simulink model "Modified_CR"  (R2014b)
settings: Solver=ode45  StartTime=0.0  StopTime=10  RelTol=1e-3
undefined symbols (not defined in the file or in its folder): A, B, C, D
settings Model: Creator=uidd7441  LastModifiedBy=uidd7441

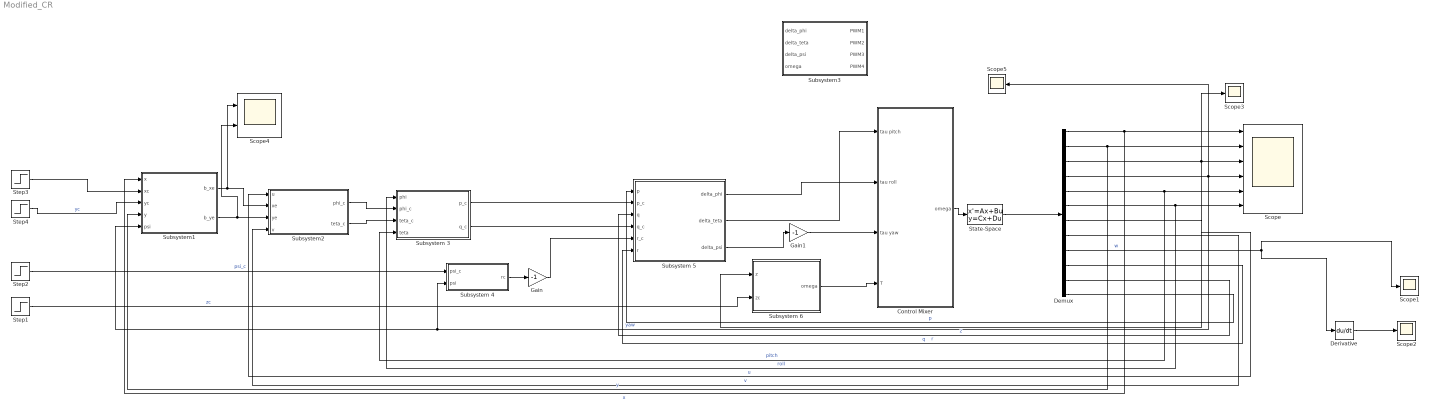
== system Modified_CR ==
  Control Mixer : Subsystem  AncestorBlock=roblocks/Dynamics/Control Mixer 4
      mask help: Quadrotor control mixer
      mask Help:
      | Determine rotor speeds based on desired torques and thrust.
      | 
      | <b>Inputs::</b>
      | 
      | tau pitch (1x1)  desired pitching torque [Nm]
      | tau roll (1x1)   desired rolling torque [Nm]
      | tau yaw (1x1)    desired yawing torque [Nm]
      | T (1x1)          desired thrust [N]
      | 
      | <b>Outputs::</b>
      | 
      | w1 (1x1) angular velocity of rotor 1 [rad]
      | w2 (1x1) angular velocity of rotor 2 [rad]
      | w3 (1x1) angular velocity of rotor 3 [rad]
      | w4 (1x1) angular velocity of rotor 4 [rad]
      | 
      | <b>Notes::</b>
      | 
      | - Assumes the rotor labelling convention of RVC Fig 4.16.
      | - The quadrotor is underactuated and has only 4 inputs.
  Demux : Demux  Outputs=12
  Derivative : Derivative
  Gain : Gain  Gain=-1
  Gain1 : Gain  Gain=-1
  Scope : Scope  NumInputPorts=6
      settings: YMin=0~0~0~0~0~-4e+06  YMax=2e+08~2e+08~1000~400000~4e+06~0
  Scope{1..3,5} (4 alike) : Scope
      Scope2 settings: SaveName=ScopeData2
      Scope3 settings: SaveName=ScopeData3
      Scope5 settings: TimeRange=2.494596015329648  YMin=250000  YMax=450000  SaveName=ScopeData5  MaxDataPoints=5000000
  Scope4 : Scope  NumInputPorts=2
      settings: YMin=-5~-5  YMax=5~5  SaveName=ScopeData10
  State-Space : StateSpace  A=A  B=B  C=C  D=D  X0=[0 0 0 0 0 0 0 0 0 0 0 0]'
  Step1 : Step  Time=0  SampleTime=0
  Step2 : Step  Time=0  After=60  SampleTime=0
  Step3 : Step  Time=0  SampleTime=0
  Step4 : Step  Time=0  SampleTime=0
  Subsystem 3 : Subsystem
  Subsystem 4 : Subsystem
  Subsystem 5 : Subsystem
  Subsystem 6 : Subsystem
  Subsystem1 : Subsystem
  Subsystem2 : Subsystem
  Subsystem3 : Subsystem
  wires:
  Step1/1 -> Subsystem 6/2(zc)  "zc"
  Step4/1 -> Subsystem1/3(yc)  "yc"
  Step2/1 -> Subsystem 4/1(psi_c)  "psi_c"
  Subsystem1/2(b_ye) -> Scope4/2, Subsystem2/3(ye)
  Subsystem 4/1(rc) -> Gain/1
  Subsystem 6/1(omega) -> Control Mixer/4(T)
  State-Space/1 -> Demux/1
  Subsystem1/1(b_xe) -> Scope4/1, Subsystem2/2(xe)
  Step3/1 -> Subsystem1/2(xc)
  Demux/3 -> Subsystem 6/1(z), Scope3/1, Scope/3  "z"
  Demux/1 -> Subsystem1/1(x), Scope/1  "x"
  Demux/2 -> Subsystem1/4(y), Scope/2  "y"
  Demux/4 -> Subsystem1/5(psi), Subsystem 4/2(psi), Scope5/1, Scope/4  "yaw"
  Demux/5 -> Subsystem 3/4(teta), Scope/5  "pitch"
  Demux/6 -> Subsystem 3/1("phi "), Scope/6  "roll"
  Demux/7 -> Subsystem2/1(u)  "u"
  Demux/8 -> Subsystem2/4(v)  "v"
  Demux/9 -> Scope1/1, Derivative/1  "w"
  Demux/11 -> Subsystem 5/3(q)  "q"
  Demux/12 -> Subsystem 5/1(p)  "p"
  Demux/10 -> Subsystem 5/6(r)  "r"
  Derivative/1 -> Scope2/1
  Subsystem 5/3(delta_psi) -> Gain1/1
  Subsystem 3/1(p_c) -> Subsystem 5/2(p_c)
  Subsystem 3/2(q_c) -> Subsystem 5/4(q_c)
  Gain/1 -> Subsystem 5/5(r_c)
  Gain1/1 -> Control Mixer/3(tau yaw)
  Control Mixer/1(omega) -> State-Space/1
  Subsystem2/1(phi_c) -> Subsystem 3/2(phi_c)
  Subsystem2/2(teta_c) -> Subsystem 3/3(teta_c)
  Subsystem 5/1(delta_phi) -> Control Mixer/2(tau roll)
  Subsystem 5/2(delta_teta) -> Control Mixer/1(tau pitch)

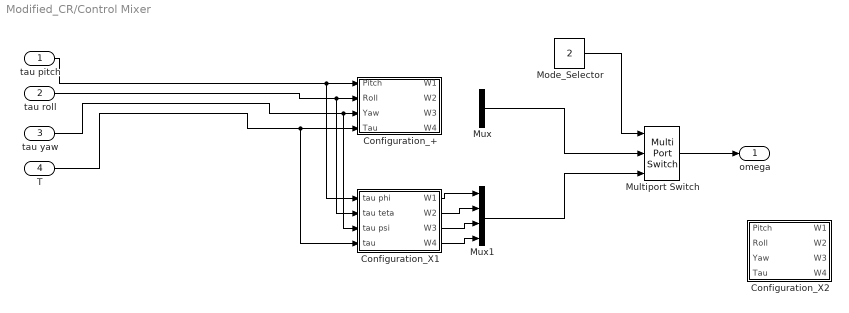
== system Modified_CR/Control Mixer ==
  tau pitch : Inport
  tau roll : Inport  Port=2
  tau yaw : Inport  Port=3
  T : Inport  Port=4
  Configuration_+ : Subsystem
  Configuration_X1 : Subsystem
  Configuration_X2 : Subsystem
  Mode_Selector : Constant  Value=2
  Multiport Switch : MultiPortSwitch  Inputs=2
  Mux : Mux
  Mux1 : Mux
  omega : Outport
  wires:
  Mux/1 -> Multiport Switch/2
  Multiport Switch/1 -> omega/1
  Mode_Selector/1 -> Multiport Switch/1
  T/1 -> Configuration_X1/4(tau), Configuration_+/4(Tau)
  tau yaw/1 -> Configuration_X1/3(tau psi), Configuration_+/3(Yaw)
  tau roll/1 -> Configuration_X1/2(tau teta), Configuration_+/2(Roll)
  tau pitch/1 -> Configuration_X1/1(tau phi), Configuration_+/1(Pitch)
  Mux1/1 -> Multiport Switch/3
  Configuration_X1/4(W4) -> Mux1/4
  Configuration_X1/3(W3) -> Mux1/3
  Configuration_X1/2(W2) -> Mux1/2
  Configuration_X1/1(W1) -> Mux1/1

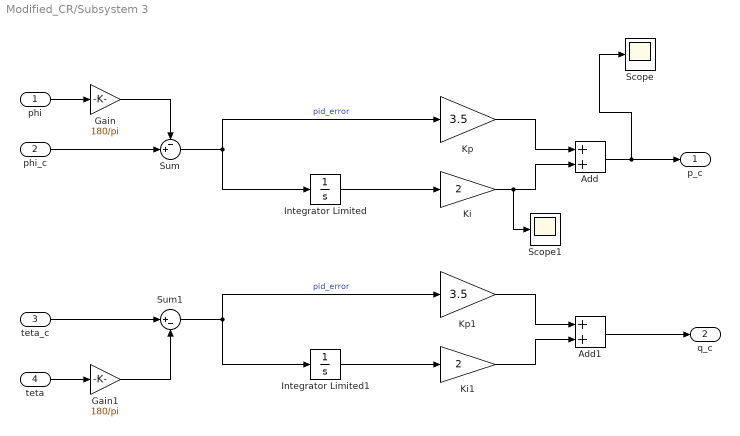
== system Modified_CR/Subsystem 3 ==
  "phi " : Inport
  phi_c : Inport  Port=2
  teta_c : Inport  Port=3
  teta : Inport  Port=4
  Add : Sum
  Add1 : Sum
  Gain : Gain  Gain=180/pi
  Gain1 : Gain  Gain=180/pi
  Integrator Limited : Integrator  LimitOutput=on  UpperSaturationLimit=20  LowerSaturationLimit=-20
  Integrator Limited1 : Integrator  LimitOutput=on  UpperSaturationLimit=20  LowerSaturationLimit=-20
  Ki : Gain  Gain=2  OutMin=[-200]  OutMax=[200]
  Ki1 : Gain  Gain=2  OutMin=[-200]  OutMax=[200]
  Kp : Gain  Gain=3.5  OutMin=[-200]  OutMax=[200]
  Kp1 : Gain  Gain=3.5  OutMin=[-200]  OutMax=[200]
  Scope : Scope
      settings: SaveName=ScopeData7
  Scope1 : Scope
      settings: SaveName=ScopeData8
  Sum : Sum  Inputs=-+|
  Sum1 : Sum  Inputs=|+-
  p_c : Outport
  q_c : Outport  Port=2
  wires:
  "phi "/1 -> Gain/1
  phi_c/1 -> Sum/2
  teta_c/1 -> Sum1/1
  teta/1 -> Gain1/1
  Add/1 -> Scope/1, p_c/1
  Add1/1 -> q_c/1
  Sum/1 -> Integrator Limited/1, Kp/1  "pid_error"
  Integrator Limited/1 -> Ki/1
  Kp/1 -> Add/1
  Sum1/1 -> Integrator Limited1/1, Kp1/1  "pid_error"
  Integrator Limited1/1 -> Ki1/1
  Kp1/1 -> Add1/1
  Ki1/1 -> Add1/2
  Gain/1 -> Sum/1
  Gain1/1 -> Sum1/2
  Ki/1 -> Scope1/1, Add/2

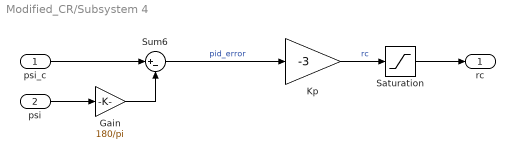
== system Modified_CR/Subsystem 4 ==
  psi_c : Inport
  psi : Inport  Port=2
  Gain : Gain  Gain=180/pi
  Kp : Gain  Gain=-3  OutMin=[-200]  OutMax=[200]
  Saturation : Saturate  UpperLimit=200  LowerLimit=-200
  Sum6 : Sum  Inputs=|+-
  rc : Outport
  wires:
  Kp/1 -> Saturation/1  "rc"
  psi_c/1 -> Sum6/1
  psi/1 -> Gain/1
  Sum6/1 -> Kp/1  "pid_error"
  Saturation/1 -> rc/1
  Gain/1 -> Sum6/2

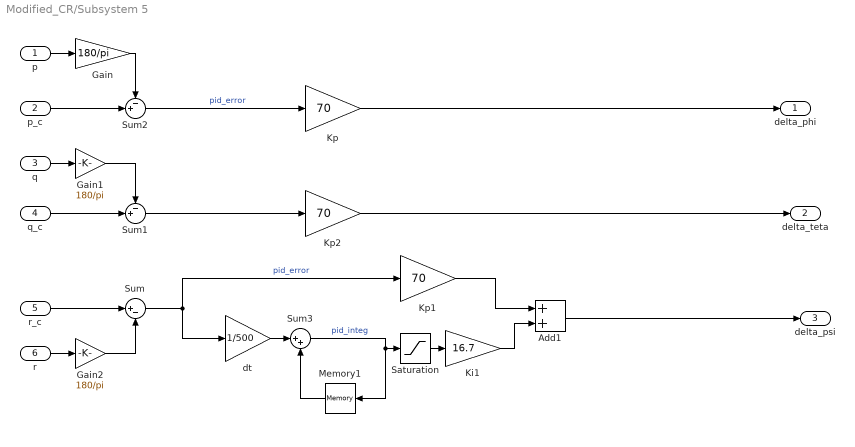
== system Modified_CR/Subsystem 5 ==
  p : Inport
  p_c : Inport  Port=2
  q : Inport  Port=3
  q_c : Inport  Port=4
  r_c : Inport  Port=5
  r : Inport  Port=6
  Add1 : Sum
  Gain : Gain  Gain=180/pi
  Gain1 : Gain  Gain=180/pi
  Gain2 : Gain  Gain=180/pi
  Ki1 : Gain  Gain=16.7  OutMin=[-200]  OutMax=[200]
  Kp : Gain  Gain=70  OutMin=[-200]  OutMax=[200]
  Kp1 : Gain  Gain=70  OutMin=[-200]  OutMax=[200]
  Kp2 : Gain  Gain=70  OutMin=[-200]  OutMax=[200]
  Memory1 : Memory
  Saturation : Saturate  UpperLimit=166.7  LowerLimit=-166.7
  Sum : Sum  Inputs=|+-
  Sum1 : Sum  Inputs=-+|
  Sum2 : Sum  Inputs=-+|
  Sum3 : Sum  Inputs=|++
  dt : Gain  Gain=1/500  OutMin=[-200]  OutMax=[200]
  delta_phi : Outport
  delta_teta : Outport  Port=2
  delta_psi : Outport  Port=3
  wires:
  q/1 -> Gain1/1
  q_c/1 -> Sum1/2
  p_c/1 -> Sum2/2
  p/1 -> Gain/1
  r_c/1 -> Sum/1
  r/1 -> Gain2/1
  Sum1/1 -> Kp2/1
  Kp/1 -> delta_phi/1
  Kp2/1 -> delta_teta/1
  Add1/1 -> delta_psi/1
  Sum2/1 -> Kp/1  "pid_error"
  Kp1/1 -> Add1/1
  Ki1/1 -> Add1/2
  dt/1 -> Sum3/1
  Sum/1 -> Kp1/1, dt/1  "pid_error"
  Sum3/1 -> Saturation/1, Memory1/1  "pid_integ"
  Memory1/1 -> Sum3/2
  Saturation/1 -> Ki1/1
  Gain/1 -> Sum2/1
  Gain1/1 -> Sum1/1
  Gain2/1 -> Sum/2

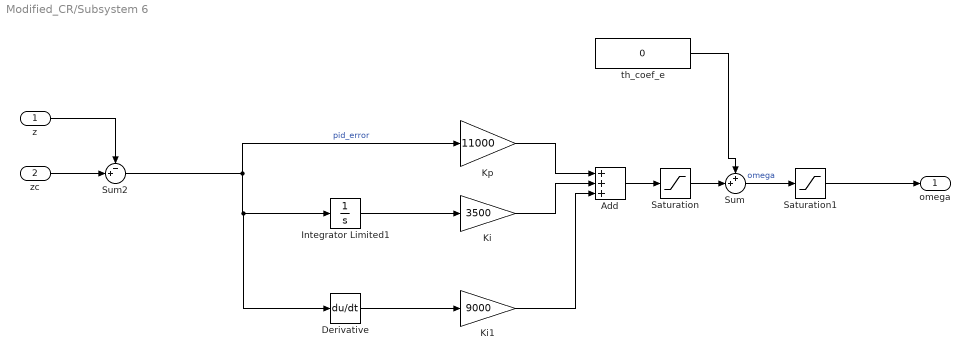
== system Modified_CR/Subsystem 6 ==
  z : Inport
  zc : Inport  Port=2
  Add : Sum  Inputs=+++
  Derivative : Derivative
  Integrator Limited1 : Integrator  LimitOutput=on  UpperSaturationLimit=1000  LowerSaturationLimit=-1000
  Ki : Gain  Gain=3500  OutMin=[-200]  OutMax=[200]
  Ki1 : Gain  Gain=9000  OutMin=[-200]  OutMax=[200]
  Kp : Gain  Gain=11000  OutMin=[-200]  OutMax=[200]
  Saturation : Saturate  UpperLimit=15000  LowerLimit=-20000
  Saturation1 : Saturate  UpperLimit=60000  LowerLimit=-20000
  Sum : Sum  Inputs=++|
  Sum2 : Sum  Inputs=-+|
  "th_coef_e " : Constant  Value=0
  omega : Outport
  wires:
  "th_coef_e "/1 -> Sum/1
  Sum/1 -> Saturation1/1  "omega"
  zc/1 -> Sum2/2
  z/1 -> Sum2/1
  Sum2/1 -> Derivative/1, Integrator Limited1/1, Kp/1  "pid_error"
  Integrator Limited1/1 -> Ki/1
  Kp/1 -> Add/1
  Ki/1 -> Add/2
  Ki1/1 -> Add/3
  Derivative/1 -> Ki1/1
  Add/1 -> Saturation/1
  Saturation/1 -> Sum/2
  Saturation1/1 -> omega/1

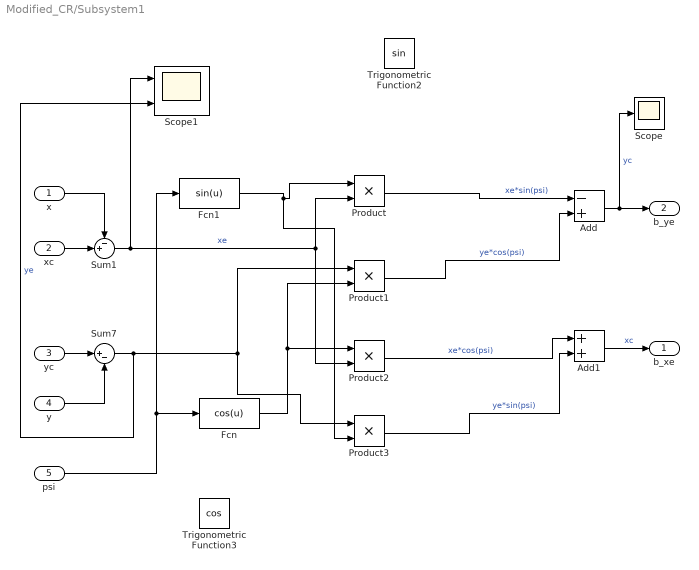
== system Modified_CR/Subsystem1 ==
  x : Inport
  xc : Inport  Port=2
  yc : Inport  Port=3
  y : Inport  Port=4
  psi : Inport  Port=5
  Add : Sum  Inputs=-+
  Add1 : Sum
  Fcn : Fcn  Expr=cos(u)
  Fcn1 : Fcn  Expr=sin(u)
  Product{,1..3} (4 alike) : Product
  Scope : Scope
      settings: SaveName=ScopeData9
  Scope1 : Scope  NumInputPorts=2
      settings: YMin=-5~-5  YMax=5~5  SaveName=ScopeData11
  Sum1 : Sum  Inputs=-+|
  Sum7 : Sum  Inputs=|+-
  Trigonometric Function2 : Trigonometry
  Trigonometric Function3 : Trigonometry  Operator=cos
  b_xe : Outport
  b_ye : Outport  Port=2
  wires:
  Sum1/1 -> Scope1/1, Product/2, Product2/2  "xe"
  Sum7/1 -> Scope1/2, Product1/1, Product3/1  "ye"
  Fcn1/1 -> Product3/2, Product/1
  Product/1 -> Add/1  "xe*sin(psi)"
  Product1/1 -> Add/2  "ye*cos(psi)"
  Fcn/1 -> Product1/2, Product2/1
  Product2/1 -> Add1/1  "xe*cos(psi)"
  Product3/1 -> Add1/2  "ye*sin(psi)"
  Add/1 -> Scope/1, b_ye/1  "yc"
  Add1/1 -> b_xe/1  "xc"
  x/1 -> Sum1/1
  xc/1 -> Sum1/2
  yc/1 -> Sum7/1
  y/1 -> Sum7/2
  psi/1 -> Fcn1/1, Fcn/1

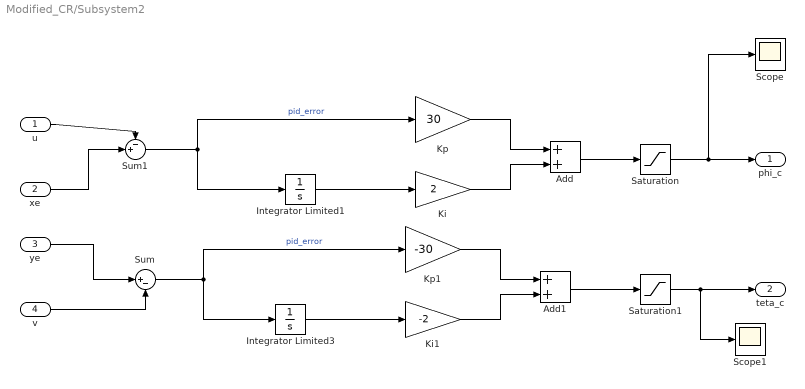
== system Modified_CR/Subsystem2 ==
  u : Inport
  xe : Inport  Port=2
  ye : Inport  Port=3
  v : Inport  Port=4
  Add : Sum
  Add1 : Sum
  Integrator Limited1 : Integrator  LimitOutput=on  UpperSaturationLimit=0.1  LowerSaturationLimit=-0.1
  Integrator Limited3 : Integrator  LimitOutput=on  UpperSaturationLimit=0.1  LowerSaturationLimit=-0.1
  Ki : Gain  Gain=2  OutMin=[-200]  OutMax=[200]
  Ki1 : Gain  Gain=-2  OutMin=[-200]  OutMax=[200]
  Kp : Gain  Gain=30  OutMin=[-200]  OutMax=[200]
  Kp1 : Gain  Gain=-30  OutMin=[-200]  OutMax=[200]
  Saturation : Saturate  UpperLimit=30  LowerLimit=-30
  Saturation1 : Saturate  UpperLimit=30  LowerLimit=-30
  Scope : Scope
      settings: SaveName=ScopeData4
  Scope1 : Scope
      settings: SaveName=ScopeData6
  Sum : Sum  Inputs=|+-
  Sum1 : Sum  Inputs=-+|
  phi_c : Outport
  teta_c : Outport  Port=2
  wires:
  u/1 -> Sum1/1
  xe/1 -> Sum1/2
  ye/1 -> Sum/1
  v/1 -> Sum/2
  Sum1/1 -> Integrator Limited1/1, Kp/1  "pid_error"
  Integrator Limited1/1 -> Ki/1
  Kp/1 -> Add/1
  Ki/1 -> Add/2
  Sum/1 -> Integrator Limited3/1, Kp1/1  "pid_error"
  Integrator Limited3/1 -> Ki1/1
  Kp1/1 -> Add1/1
  Ki1/1 -> Add1/2
  Add1/1 -> Saturation1/1
  Add/1 -> Saturation/1
  Saturation/1 -> Scope/1, phi_c/1
  Saturation1/1 -> Scope1/1, teta_c/1

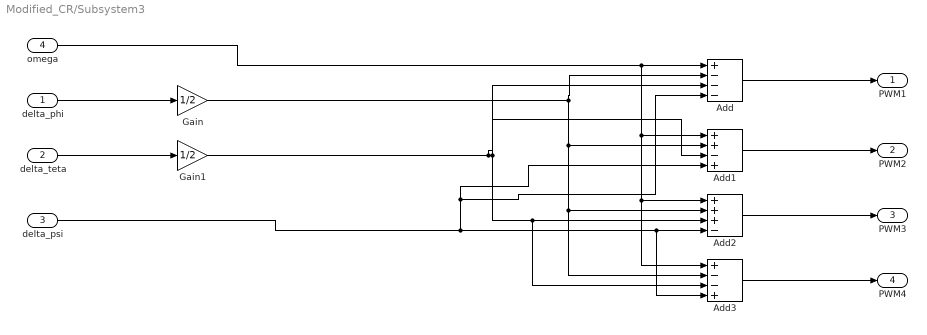
== system Modified_CR/Subsystem3 ==
  delta_phi : Inport
  delta_teta : Inport  Port=2
  delta_psi : Inport  Port=3
  omega : Inport  Port=4
  Add : Sum  Inputs=+---
  Add1 : Sum  Inputs=++-+
  Add2 : Sum  Inputs=+++-
  Add3 : Sum  Inputs=+--+
  Gain : Gain  Gain=1/2
  Gain1 : Gain  Gain=1/2
  PWM1 : Outport
  PWM2 : Outport  Port=2
  PWM3 : Outport  Port=3
  PWM4 : Outport  Port=4
  wires:
  Gain1/1 -> Add/3, Add2/3, Add3/3, Add1/3
  Gain/1 -> Add2/2, Add3/2, Add1/2, Add/2
  delta_psi/1 -> Add/4, Add1/4, Add2/4, Add3/4
  omega/1 -> Add/1, Add1/1, Add2/1, Add3/1
  Add3/1 -> PWM4/1
  Add2/1 -> PWM3/1
  Add1/1 -> PWM2/1
  Add/1 -> PWM1/1
  delta_teta/1 -> Gain1/1
  delta_phi/1 -> Gain/1

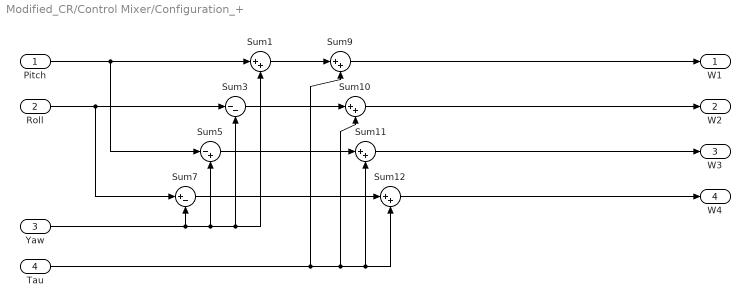
== system Modified_CR/Control Mixer/Configuration_+ ==
  Pitch : Inport
  Roll : Inport  Port=2
  Yaw : Inport  Port=3
  Tau : Inport  Port=4
  Sum{1,9..12} (5 alike) : Sum  Inputs=|++  SaturateOnIntegerOverflow=on  InputSameDT=on  OutDataTypeStr=Inherit: Same as first input
  Sum3 : Sum  Inputs=|--  SaturateOnIntegerOverflow=on  InputSameDT=on  OutDataTypeStr=Inherit: Same as first input
  Sum5 : Sum  Inputs=|-+  SaturateOnIntegerOverflow=on  InputSameDT=on  OutDataTypeStr=Inherit: Same as first input
  Sum7 : Sum  Inputs=|+-  SaturateOnIntegerOverflow=on  InputSameDT=on  OutDataTypeStr=Inherit: Same as first input
  W1 : Outport
  W2 : Outport  Port=2
  W3 : Outport  Port=3
  W4 : Outport  Port=4
  wires:
  Sum3/1 -> Sum10/1
  Sum1/1 -> Sum9/1
  Sum10/1 -> W2/1
  Sum7/1 -> Sum12/1
  Sum12/1 -> W4/1
  Sum11/1 -> W3/1
  Roll/1 -> Sum7/1, Sum3/1
  Pitch/1 -> Sum5/1, Sum1/1
  Sum9/1 -> W1/1
  Tau/1 -> Sum9/2, Sum10/2, Sum12/2, Sum11/2
  Yaw/1 -> Sum1/2, Sum3/2, Sum5/2, Sum7/2
  Sum5/1 -> Sum11/1

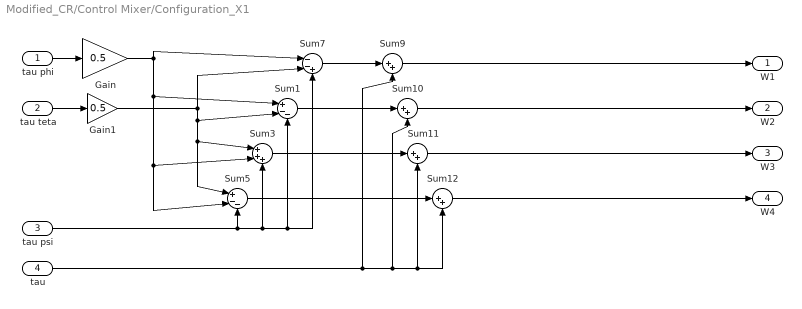
== system Modified_CR/Control Mixer/Configuration_X1 ==
  tau phi : Inport
  tau teta : Inport  Port=2
  tau psi : Inport  Port=3
  tau : Inport  Port=4
  Gain : Gain  Gain=0.5
  Gain1 : Gain  Gain=0.5
  Sum1 : Sum  Inputs=|+--  SaturateOnIntegerOverflow=on  InputSameDT=on  OutDataTypeStr=Inherit: Same as first input
  Sum{9..12} (4 alike) : Sum  Inputs=|++  SaturateOnIntegerOverflow=on  InputSameDT=on  OutDataTypeStr=Inherit: Same as first input
  Sum3 : Sum  Inputs=|+++  SaturateOnIntegerOverflow=on  InputSameDT=on  OutDataTypeStr=Inherit: Same as first input
  Sum5 : Sum  Inputs=|+--  SaturateOnIntegerOverflow=on  InputSameDT=on  OutDataTypeStr=Inherit: Same as first input
  Sum7 : Sum  Inputs=|--+  SaturateOnIntegerOverflow=on  InputSameDT=on  OutDataTypeStr=Inherit: Same as first input
  W1 : Outport
  W2 : Outport  Port=2
  W3 : Outport  Port=3
  W4 : Outport  Port=4
  wires:
  Sum12/1 -> W4/1
  Sum11/1 -> W3/1
  Sum10/1 -> W2/1
  Sum9/1 -> W1/1
  Gain1/1 -> Sum3/1, Sum5/1, Sum1/2, Sum7/2
  Gain/1 -> Sum3/2, Sum5/2, Sum1/1, Sum7/1
  tau phi/1 -> Gain/1
  tau teta/1 -> Gain1/1
  Sum1/1 -> Sum10/1
  Sum7/1 -> Sum9/1
  Sum5/1 -> Sum12/1
  tau/1 -> Sum9/2, Sum10/2, Sum12/2, Sum11/2
  tau psi/1 -> Sum1/3, Sum7/3, Sum3/3, Sum5/3
  Sum3/1 -> Sum11/1

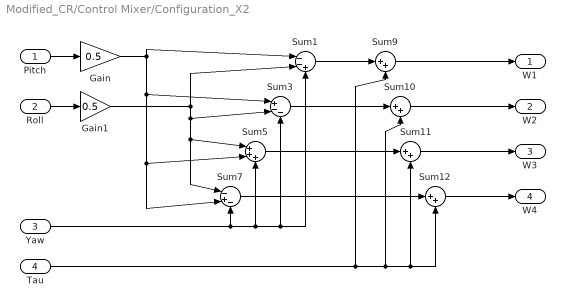
== system Modified_CR/Control Mixer/Configuration_X2 ==
  Pitch : Inport
  Roll : Inport  Port=2
  Yaw : Inport  Port=3
  Tau : Inport  Port=4
  Gain : Gain  Gain=0.5
  Gain1 : Gain  Gain=0.5
  Sum1 : Sum  Inputs=|--+  SaturateOnIntegerOverflow=on  InputSameDT=on  OutDataTypeStr=Inherit: Same as first input
  Sum{9..12} (4 alike) : Sum  Inputs=|++  SaturateOnIntegerOverflow=on  InputSameDT=on  OutDataTypeStr=Inherit: Same as first input
  Sum3 : Sum  Inputs=|+--  SaturateOnIntegerOverflow=on  InputSameDT=on  OutDataTypeStr=Inherit: Same as first input
  Sum5 : Sum  Inputs=|+++  SaturateOnIntegerOverflow=on  InputSameDT=on  OutDataTypeStr=Inherit: Same as first input
  Sum7 : Sum  Inputs=|-+-  SaturateOnIntegerOverflow=on  InputSameDT=on  OutDataTypeStr=Inherit: Same as first input
  W1 : Outport
  W2 : Outport  Port=2
  W3 : Outport  Port=3
  W4 : Outport  Port=4
  wires:
  Sum5/1 -> Sum11/1
  Yaw/1 -> Sum7/3, Sum5/3, Sum1/3, Sum3/3
  Tau/1 -> Sum11/2, Sum12/2, Sum10/2, Sum9/2
  Sum7/1 -> Sum12/1
  Sum1/1 -> Sum9/1
  Sum3/1 -> Sum10/1
  Roll/1 -> Gain1/1
  Pitch/1 -> Gain/1
  Gain/1 -> Sum3/1, Sum7/2, Sum5/2, Sum1/1
  Gain1/1 -> Sum1/2, Sum3/2, Sum5/1, Sum7/1
  Sum9/1 -> W1/1
  Sum10/1 -> W2/1
  Sum11/1 -> W3/1
  Sum12/1 -> W4/1
